simulink model "Simulink_Simulation"  (Simulink 10.1)
settings: Solver=ode23t  StartTime=0.0  StopTime=0.1  RelTol=1e-3  EnableMultiTasking=on
libraries: powerlib x11, powerlib_meascontrol x4
settings Model: Creator=asus1  LastModifiedBy=x64
settings DataIOCC: LimitDataPoints=on
settings DebuggingCC: UnderspecifiedInitializationDetection=Simplified  MergeDetectMultiDrivingBlocksExec=error  SolverPrmCheckMsg=warning
settings GRTTargetCC: CombineOutputUpdateFcns=on  GRTInterface=off
settings ConfigComp: CovSFcnEnable=off
settings SimscapeCC: SimscapeNormalizeSystem=off

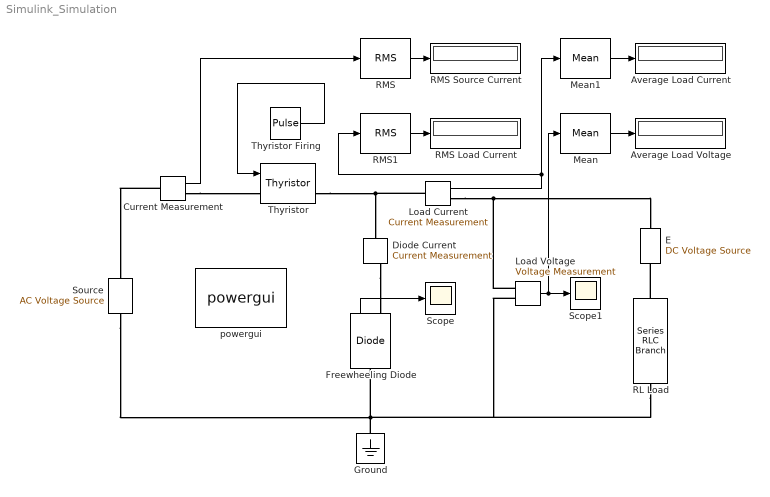
== system Simulink_Simulation ==
  Average Load Current : Display
      settings: Format=bank
  Average Load Voltage : Display
      settings: Format=bank
  Current Measurement : powerlib/Measurements/Current Measurement  PhasorSimulation=off  OutputType=Complex  PSBequivalent=0
  Diode Current : powerlib/Measurements/Current Measurement  PhasorSimulation=off  OutputType=Complex  PSBequivalent=0
  E : powerlib/Electrical Sources/DC Voltage Source  Amplitude=220  Measurements=None
  Freewheeling Diode : powerlib/Power Electronics/Diode  Ron=0.00000001  Lon=0  Vf=0  IC=0  UseSnubber=off  Rs=5000  Cs=250e-9  Measurements=on
  Ground : powerlib/Elements/Ground  LConnTagsString=a
  Load Current : powerlib/Measurements/Current Measurement  PhasorSimulation=off  OutputType=Complex  PSBequivalent=0
  Load Voltage : powerlib/Measurements/Voltage Measurement  PhasorSimulation=off  OutputType=Complex  PSBequivalent=0
  Mean : powerlib_meascontrol/Measurements/Mean  Freq=50  Vinit=0  Ts=0
  Mean1 : powerlib_meascontrol/Measurements/Mean  Freq=50  Vinit=0  Ts=0
  RL Load : powerlib/Elements/Series RLC Branch  LConnTagsString=__new0  RConnTagsString=__new0  BranchType=RL  Resistance=1  Inductance=0.01  SetiL0=off  InitialCurrent=0  Capacitance=1e-6  Setx0=off  InitialVoltage=0  Measurements=None
  RMS : powerlib_meascontrol/Measurements/RMS  TrueRMS=on  Freq=50  RMSInit=120  Ts=0
  RMS Load Current : Display
      settings: Format=bank
  RMS Source Current : Display
      settings: Format=bank
  RMS1 : powerlib_meascontrol/Measurements/RMS  TrueRMS=on  Freq=50  RMSInit=120  Ts=0
  Scope : Scope
  Scope1 : Scope
  Source : powerlib/Electrical Sources/AC Voltage Source  Amplitude=220*sqrt(2)  Phase=0  Frequency=50  SampleTime=0  Measurements=None  BusType=swing  Pref=10e3  Qref=0  Qmin=-inf  Qmax=+inf
  "Thyristor " : powerlib/Power Electronics/Thyristor  Ron=0.0000001  Lon=0  Vf=0  IC=0  Rs=5000  Cs=250e-9  Measurements=on
  "Thyristor Firing " : DiscretePulseGenerator  PulseType=Time based  Period=0.02  PulseWidth=50  PhaseDelay=(90/360)*0.02
  powergui : powerlib/powergui  Priority=1  SimulationMode=Discrete  SampleTime=50e-7  frequency=60  Iterations=50  frequencyindice=50  Pbase=100e6  ErrMax=1e-4  UnitsV=kV  UnitsW=MW  buscounter=0  FunctionMessages=off  echomessages=off  EnableUseOfTLC=off  CurrentSourceSwitches=off  DisableSnubberDevices=off  DisableRonSwitches=off  DisableVfSwitches=off  DisplayEquations=off  AutomaticDiscreteSolvers=off  SolverType=Tustin  Interpol=off  ExternalGateDelay=off  methode=off  Ts=100  x0status=blocks  SPID=off  SwTol=0  HookPort=off  NonlinearTolerance=1e-4  nMaxIteration=100  ContinueOnMaxIteration=off  RestoreLinks=warning  ResistiveCurrentMeasurement=off  Frange=[0:2:500]  Ylog=off  Xlog=on  ShowGrid=off  save=off  variable=ZData  structure=0  ZoomFFT=off  StartTime=0.0  cycles=1  DisplayStyle=1  fundamental=60  FreqAxis=off  MaxFrequency=1000  frequencyindicesteady=1  RmsSteady=1  display=off
  wires:
  "Thyristor Firing "/1 -> "Thyristor "/1
  RMS/1 -> RMS Source Current/1
  RMS1/1 -> RMS Load Current/1
  Mean1/1 -> Average Load Current/1
  Mean/1 -> Average Load Voltage/1
  Freewheeling Diode/1 -> Scope/1
  Load Voltage/1 -> Mean/1, Scope1/1
  Current Measurement/1 -> RMS/1
  Load Current/1 -> Mean1/1, RMS1/1
  connections:
  Current Measurement/RConn1 -- "Thyristor "/LConn1
  Current Measurement/LConn1 -- Source/RConn1
  "Thyristor "/RConn1 -- Load Current/LConn1 -- Diode Current/LConn1
  Diode Current/RConn1 -- Freewheeling Diode/RConn1
  Source/LConn1 -- Load Voltage/LConn2 -- RL Load/RConn1 -- Ground/LConn1 -- Freewheeling Diode/LConn1
  Load Current/RConn1 -- E/RConn1 -- Load Voltage/LConn1
  RL Load/LConn1 -- E/LConn1
